simulink model "SimulacaoSIR"  (R2021b)
settings: Solver=VariableStepAuto  StartTime=0.0  StopTime=1000  RelTol=1e-3
values from neighbouring files (symbols this model uses):
  beta = X(1)    [ErroQuadratico.m]
  i0 = 1    [ErroQuadratico.m]
  r = X(2)    [ErroQuadratico.m]
  r0 = 0    [ErroQuadratico.m]
  s0 = N - i0    (= 499)    [ErroQuadratico.m]
settings Model: Creator=20.01937-8  LastModifiedBy=STORM
settings SolverCC: AlgebraicLoopSolver=TrustRegion
settings DataIOCC: ReturnWorkspaceOutputs=off
settings DebuggingCC: SFMachineParentedDataDiag=warning  ArithmeticOperatorsInVariantConditions=warning
settings SFSimCC: CustomCodeUndefinedFunction=UseInterfaceOnly

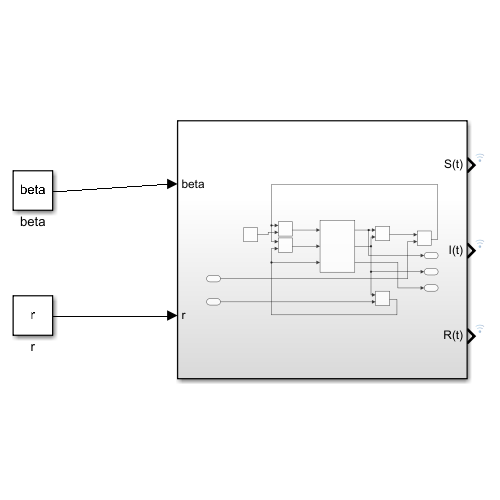
[thumbnail: Simulink's stored preview of the top-level diagram]
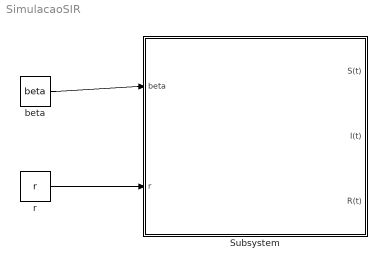
== system SimulacaoSIR ==
  Subsystem : Subsystem
  "beta " : Constant  Value=beta
  r : Constant  Value=r
  wires:
  "beta "/1 -> Subsystem/1(beta)
  r/1 -> Subsystem/2(r)

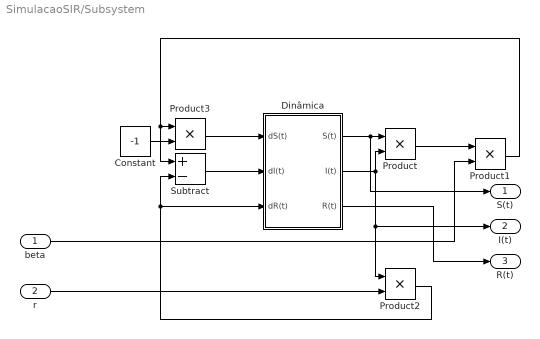
== system SimulacaoSIR/Subsystem ==
  beta : Inport
  r : Inport  Port=2
  Constant : Constant  Value=-1
  Dinâmica : Subsystem
  Product{,1..3} (4 alike) : Product
  Subtract : Sum  Inputs=+-
  S(t) : Outport  SampleTime=1.001  VectorParamsAs1DForOutWhenUnconnected=off
  I(t) : Outport  Port=2  SampleTime=1.001  VectorParamsAs1DForOutWhenUnconnected=off
  R(t) : Outport  Port=3  SampleTime=1.001  VectorParamsAs1DForOutWhenUnconnected=off
  wires:
  Dinâmica/1(S(t)) -> S(t)/1, Product/1
  Product/1 -> Product1/1
  beta/1 -> Product1/2
  Product3/1 -> Dinâmica/1(dS(t))
  Subtract/1 -> Dinâmica/2(dI(t))
  Dinâmica/2(I(t)) -> I(t)/1, Product2/1, Product/2
  Product1/1 -> Subtract/1, Product3/1
  Constant/1 -> Product3/2
  Product2/1 -> Subtract/2, Dinâmica/3(dR(t))
  Dinâmica/3(R(t)) -> R(t)/1
  r/1 -> Product2/2

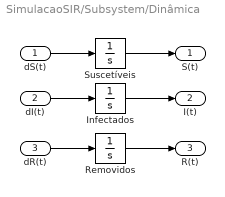
== system SimulacaoSIR/Subsystem/Dinâmica ==
  dS(t) : Inport
  dI(t) : Inport  Port=2
  dR(t) : Inport  Port=3
  Infectados : Integrator  InitialCondition=i0
  Removidos : Integrator  InitialCondition=r0
  Suscetíveis : Integrator  InitialCondition=s0
  S(t) : Outport  VectorParamsAs1DForOutWhenUnconnected=off
  I(t) : Outport  Port=2  VectorParamsAs1DForOutWhenUnconnected=off
  R(t) : Outport  Port=3  VectorParamsAs1DForOutWhenUnconnected=off
  wires:
  dS(t)/1 -> Suscetíveis/1
  Infectados/1 -> I(t)/1
  Suscetíveis/1 -> S(t)/1
  dI(t)/1 -> Infectados/1
  dR(t)/1 -> Removidos/1
  Removidos/1 -> R(t)/1
